simulink library "vehicleMMAdd"  (R2018b)
settings: Solver=VariableStepAuto  StartTime=0.0  StopTime=10.0  RelTol=1e-3
undefined symbols (not defined in the file): env, vhcl
libraries: vrlib x1, eulAng2RotMat_ul x1, dragTurbine_ul x1, fluidDynamicSurface_cl x1, sixDoFDynamics_ul x1, tethersMoment_cl x1, thrAttachPtKinematics_ul x1
settings Model: Creator=mcobb  LastModifiedBy=jldanie5

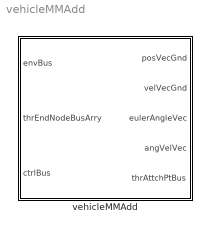
== system vehicleMMAdd ==
  vehicleMMAdd : Subsystem  VariantControl=VSS_vehicle_vehicle000  mask{vcl=vhcl, rho=env.water.density.Value, grav=env.gravAccel.Value}
      mask prompts: vcl "Vehicle"; rho "Density"; grav "Gravity"
      mask DialogControl Container9 Prompt: General
      mask DialogControl Container5 Prompt: Vehicle object (OCT.vehicle)
      mask DialogControl ParameterGroupVar Prompt: Environment Object (OCT.env)
      mask Display:
      | image('kite.jpg',[100 100 601 528]/4,'on')
      | 
      | port_label('input',1,'ctrlBus')
      | port_label('input',2,'envBus')
      | port_label('input',3,'thrEndNodeBusArry')
      | 
      | port_label('output',1,'posVecGnd')
      | port_label('output',2,'velVecGnd')
      | port_label('output',3,'eulAng')
      | port_label('output',4,'angVelVec')
      | port_label('output',5,'thrAttchPtBus')

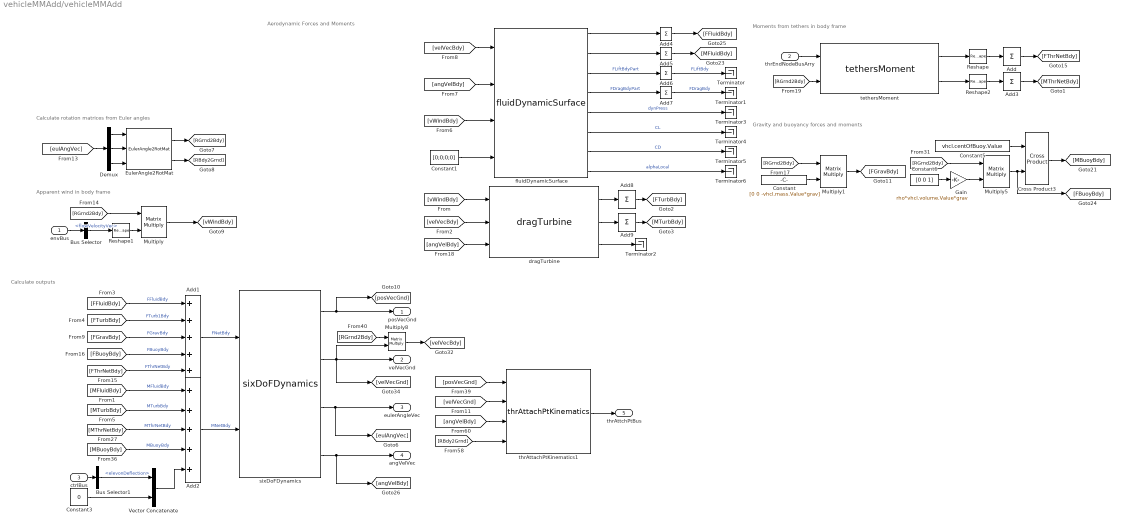
== system vehicleMMAdd/vehicleMMAdd ==
  note: Calculate outputs
  note: Apparent wind in body frame
  note: Calculate rotation matrices from Euler angles
  note: Gravity and buoyancy forces and moments
  note: Moments from tethers in body frame
  note: Aerodynamic Forces and Moments
  envBus : Inport  OutDataTypeStr=Bus: envBus
  thrEndNodeBusArry : Inport  Port=2
  ctrlBus : Inport  Port=3  OutDataTypeStr=Bus: ctrlBus
  Add : Sum  Inputs=+  CollapseMode=Specified dimension  CollapseDim=2
  Add1 : Sum  Inputs=+++++
  Add2 : Sum  Inputs=+++++
  Add3 : Sum  Inputs=+  CollapseMode=Specified dimension  CollapseDim=2
  Add{4..9} (6 alike) : Sum  Inputs=1  CollapseMode=Specified dimension  CollapseDim=2
  Bus Selector : BusSelector  OutputSignals=flowVelocityVec
  Bus Selector1 : BusSelector  OutputSignals=elevonDeflection
  Constant : Constant  Value=[0 0 -vhcl.mass.Value*grav]
  Constant1 : Constant  Value=[0;0;0;0]
  Constant3 : Constant  Value=0
  Constant5 : Constant  Value=vhcl.centOfBuoy.Value
  Constant6 : Constant  Value=[0 0 1]
  Cross Product3 : vrlib/Utilities/Cross Product
      settings: SourceProductBaseCode=VR
  Demux : Demux  Outputs=3
  EulerAngle2RotMat : eulAng2RotMat_ul/EulerAngle2RotMat  SystemSampleTime=-1
  Gain : Gain  Gain=rho*vhcl.volume.Value*grav
  Multiply{,1,5,8} (4 alike) : Product  Multiplication=Matrix(*)
  Reshape : Reshape  OutputDimensionality=Customize  OutputDimensions=[3 vhcl.numTethers.Value]
  Reshape1 : Reshape  OutputDimensionality=Column vector (2-D)
  Reshape2 : Reshape  OutputDimensionality=Customize  OutputDimensions=[3 vhcl.numTethers.Value]
  Terminator{,1..6} (7 alike) : Terminator
  Vector Concatenate : Concatenate
  dragTurbine : dragTurbine_ul/dragTurbine  rho_fluid=env.water.density.Value  turb_struct=vhcl.struct('OCT.turb')
  fluidDynamicSurface : fluidDynamicSurface_cl/fluidDynamicSurface  aeroStruct=vcl.struct('OCT.aeroSurf')  fluidDensity=env.water.density.Value
  sixDoFDynamics : sixDoFDynamics_ul/sixDoFDynamics  M=vhcl.mass.Value  J=vhcl.inertia.Value  initPos=vhcl.initPosVecGnd.Value  initVel=vhcl.initVelVecGnd.Value  initEulAngs=vhcl.initEulAngBdy.Value  initAngVel=vhcl.initAngVelVecBdy.Value
  tethersMoment : tethersMoment_cl/tethersMoment  arms=vhcl.struct('OCT.thrAttch')
  thrAttachPtKinematics1 : thrAttachPtKinematics_ul/thrAttachPtKinematics  atchPts=vhcl.struct('OCT.thrAttch')
  posVecGnd : Outport
  velVecGnd : Outport  Port=2
  eulerAngleVec : Outport  Port=3
  angVelVec : Outport  Port=4
  thrAttchPtBus : Outport  Port=5
  wires:
  Bus Selector/1 -> Reshape1/1  "<flowVelocityVec>"
  [eulAngVec] -> Demux/1
  Demux/2 -> EulerAngle2RotMat/2
  Demux/1 -> EulerAngle2RotMat/1
  Demux/3 -> EulerAngle2RotMat/3
  EulerAngle2RotMat/1 -> [RGrnd2Bdy]
  EulerAngle2RotMat/2 -> [RBdy2Grnd]
  [RGrnd2Bdy] -> Multiply/1
  Multiply/1 -> [vWindBdy]
  [RGrnd2Bdy] -> Multiply1/1
  Multiply1/1 -> [FGravBdy]
  thrEndNodeBusArry/1 -> tethersMoment/1
  Constant6/1 -> Gain/1
  Multiply5/1 -> Cross Product3/2, [FBuoyBdy]
  [RGrnd2Bdy] -> Multiply5/1
  Cross Product3/1 -> [MBuoyBdy]
  Constant5/1 -> Cross Product3/1
  [MFluidBdy] -> Add2/1  "MFluidBdy"
  [MThrNetBdy] -> Add2/3  "MThrNetBdy"
  [MTurbBdy] -> Add2/2  "MTurbBdy"
  Add2/1 -> sixDoFDynamics/2  "MNetBdy"
  sixDoFDynamics/3 -> [eulAngVec], eulerAngleVec/1
  sixDoFDynamics/4 -> [angVelBdy], angVelVec/1
  [FFluidBdy] -> Add1/1  "FFluidBdy"
  [FTurbBdy] -> Add1/2  "FTurb1Bdy"
  Constant/1 -> Multiply1/2
  fluidDynamicSurface/2 -> Add5/1
  sixDoFDynamics/1 -> [posVecGnd], posVecGnd/1
  Multiply8/1 -> [velVecBdy]
  sixDoFDynamics/2 -> velVecGnd/1, Multiply8/2, [velVecGnd]
  [RGrnd2Bdy] -> Multiply8/1
  [angVelBdy] -> thrAttachPtKinematics1/3
  thrAttachPtKinematics1/1 -> thrAttchPtBus/1
  [posVecGnd] -> thrAttachPtKinematics1/1
  [RBdy2Grnd] -> thrAttachPtKinematics1/4
  [velVecGnd] -> thrAttachPtKinematics1/2
  tethersMoment/1 -> Reshape/1
  Reshape/1 -> Add/1
  Add/1 -> [FThrNetBdy]
  [RGrnd2Bdy] -> tethersMoment/2
  Reshape1/1 -> Multiply/2
  Add3/1 -> [MThrNetBdy]
  Reshape2/1 -> Add3/1
  tethersMoment/2 -> Reshape2/1
  Add1/1 -> sixDoFDynamics/1  "FNetBdy"
  envBus/1 -> Bus Selector/1
  fluidDynamicSurface/1 -> Add4/1
  fluidDynamicSurface/3 -> Add6/1  "FLiftBdyPart"
  fluidDynamicSurface/4 -> Add7/1  "FDragBdyPart"
  [vWindBdy] -> fluidDynamicSurface/3
  [angVelBdy] -> fluidDynamicSurface/2
  [velVecBdy] -> fluidDynamicSurface/1
  Add4/1 -> [FFluidBdy]
  Add5/1 -> [MFluidBdy]
  Add6/1 -> Terminator/1  "FLiftBdy"
  Add7/1 -> Terminator1/1  "FDragBdy"
  dragTurbine/1 -> Add8/1
  dragTurbine/2 -> Add9/1
  Add8/1 -> [FTurbBdy]
  Add9/1 -> [MTurbBdy]
  dragTurbine/3 -> Terminator2/1
  [vWindBdy] -> dragTurbine/1
  [velVecBdy] -> dragTurbine/2
  [angVelBdy] -> dragTurbine/3
  [MBuoyBdy] -> Add2/4  "MBuoyBdy"
  [FThrNetBdy] -> Add1/5  "FThrNetBdy"
  [FBuoyBdy] -> Add1/4  "FBuoyBdy"
  [FGravBdy] -> Add1/3  "FGravBdy"
  Gain/1 -> Multiply5/2
  fluidDynamicSurface/5 -> Terminator3/1  "dynPress"
  fluidDynamicSurface/7 -> Terminator5/1  "CD"
  fluidDynamicSurface/6 -> Terminator4/1  "CL"
  fluidDynamicSurface/8 -> Terminator6/1  "alphaLocal"
  Constant1/1 -> fluidDynamicSurface/4
  ctrlBus/1 -> Bus Selector1/1
  Vector Concatenate/1 -> Add2/5
  Bus Selector1/1 -> Vector Concatenate/1  "<elevonDeflection>"
  Constant3/1 -> Vector Concatenate/2
